simulink model "plant2MRUE"  (R2023b)
settings: Solver=VariableStepAuto  StartTime=0.0  StopTime=7  RelTol=1e-3
model workspace (MATLAB code in the model file):
  | %% Paramètres du Système
  | % Masses
  | mw=0.1;
  | mb=1;
  | Ms=1.2;
  | 
  | % Distances
  | rho=0.07;
  | l=0.02;
  | d=0.015; % distance A-C
  | 
  | % Electriques
  | L=2.3e-3;
  | R=2.2;
  | % r;
  | 
  | % Couples
  | k=0.342;
  | 
  | % Moments inertie A TROUVER
  | Iwy=2.45e-4;
  | Ipsi=1.53e-2;
  | 
  | % Constantes utilitaires
  | beta = (Ms + 2*Iwy/rho^2);
  | gamma = Ipsi + mb*d^2;
  | alpha = 2/rho;
  | eta = l/rho;
  | 
  | %% Trajectoire d'équilibre
  | % Mouvement Rectiligne Uniforme selon axe x du laboratoire.
  | % On néglige les perturbations sur les entrées et les mesures.
  | 
  | % Références
  | ur = 1; %m/s
  | psir = 0;
  | 
  | % On fait le changement right,left (r,l) -> sum,dif (s,d)
  | % Somme des tensions gauche et droite
  | % Le "s" signifie "sum", on trouvera aussi "d"
  | % pour "difference"
  | Usbar = 2*k/rho*ur; % should not be >12V
  | 
  | Urbar = Usbar/2;
  | Ulbar = Usbar/2;
  | 
  | pbar = 0; % normally, should equals ubar*t,
  | % but is not in state function, so any value fits.
  | ubar = ur;
  | psibar = psir;
  | vbar = 0;
  | Isbar = 0;
  | Idbar = 0;
  | ybar = 0;
  | 
  | statebar = [pbar; ubar; psibar; vbar; Isbar; Idbar; ybar];
settings Model: Creator=Jules  LastModifiedBy=Jules

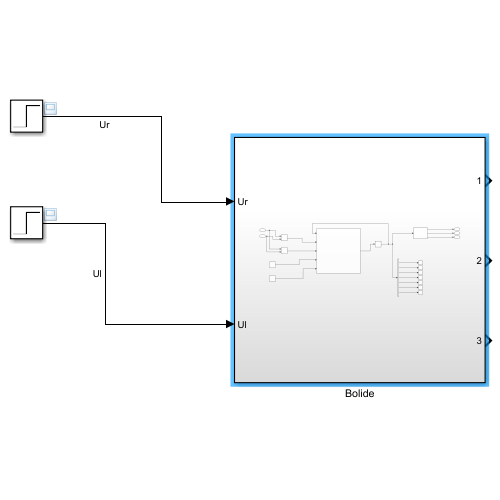
[thumbnail: Simulink's stored preview of the top-level diagram]
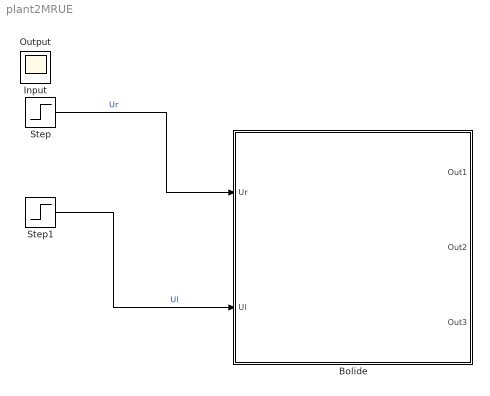
== system plant2MRUE ==
  Bolide : Subsystem
  Step : Step  Time=2  Before=Urbar  After=Urbar  SampleTime=0
  Step1 : Step  Time=2  Before=Ulbar  After=Ulbar  SampleTime=0
  Input : Scope
  Output : Scope
  wires:
  Step1/1 -> Bolide/2(Ul)  "Ul"
  Step/1 -> Bolide/1(Ur)  "Ur"

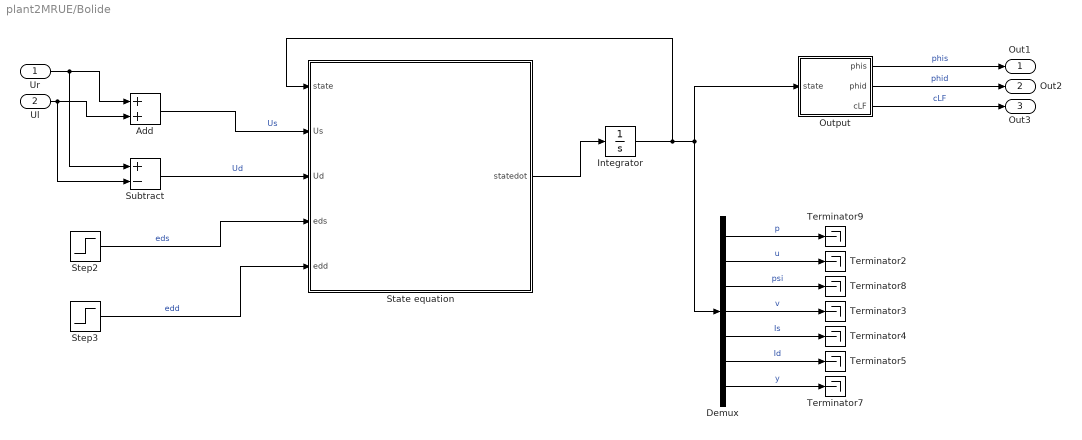
== system plant2MRUE/Bolide ==
  Ur : Inport
  Ul : Inport  Port=2
  Add : Sum
  Demux : Demux  Outputs=7
  Integrator : Integrator  InitialCondition=statebar
  Output : MATLAB Function  TreatAsAtomicUnit=on
  State equation : MATLAB Function  TreatAsAtomicUnit=on
  Step2 : Step  After=0  SampleTime=0
  Step3 : Step  After=0  SampleTime=0
  Subtract : Sum  Inputs=+-
  Terminator{2..5,7..9} (7 alike) : Terminator
  Out1 : Outport
  Out2 : Outport  Port=2
  Out3 : Outport  Port=3
  wires:
  Step3/1 -> State equation/5(edd)  "edd"
  State equation/1(statedot) -> Integrator/1
  Step2/1 -> State equation/4(eds)  "eds"
  Ul/1 -> Subtract/2, Add/2
  Ur/1 -> Subtract/1, Add/1
  Demux/1 -> Terminator9/1  "p"
  Demux/7 -> Terminator7/1  "y"
  Demux/2 -> Terminator2/1  "u"
  Demux/6 -> Terminator5/1  "Id"
  Demux/4 -> Terminator3/1  "v"
  Demux/5 -> Terminator4/1  "Is"
  Demux/3 -> Terminator8/1  "psi"
  Add/1 -> State equation/2(Us)  "Us"
  Subtract/1 -> State equation/3(Ud)  "Ud"
  Integrator/1 -> Output/1(state), Demux/1, State equation/1(state)
  Output/1(phis) -> Out1/1  "phis"
  Output/2(phid) -> Out2/1  "phid"
  Output/3(cLF) -> Out3/1  "cLF"

== matlab function plant2MRUE/Bolide/State equation ==
  data: state input; statedot output; Us input; Ud input; eds input; edd input; beta parameter; gamma parameter; rho parameter; l parameter; d parameter; L parameter; R parameter; k parameter; mb parameter
function statedot = fcn(state, Us, Ud, eds, edd, beta, gamma, rho, l, d, L, R, k, mb)
% ed est l'entrée de perturbation, != d (distance AC)
% Model parameters defined in "Model Explorer/Matlab Code"

p = state(1); % intégrale temporelle de u, distance parcourue
u = state(2);
psi = state(3);
v = state(4); % psidot
Is = state(5); % Intensité à gauche
Id = state(6);
y = state(7); % abscisse point A

pdot = u;
udot = 1/beta*(k/rho*Is - mb*d*v^2);
psidot = v;
vdot = 1/gamma*(l*k/(2*rho)*Id + mb*d*u*v);
Isdot = 1/L*((Us + eds) - R*Is - 2*k/rho*u);
Iddot = 1/L*((Ud + edd) - R*Id - k*l/rho*v);
ydot = sin(psi)*u;

statedot = [pdot; udot; psidot; vdot; Isdot; Iddot; ydot];

== matlab function plant2MRUE/Bolide/Output ==
  data: state input; alpha parameter; phis output; phid output; cLF output; eta parameter
function [phis, phid, cLF] = fcn(state,alpha,eta)
% Sorties mesurées

p = state(1);
psi = state(3);
y = state(7);

phis = alpha*p;
phid = eta*psi;
cLF = y;
